simulink model "equations_PWSM"  (R2024b)
settings: Solver=VariableStepAuto  StartTime=0.0  StopTime=10.0  RelTol=1e-3
undefined symbols (not defined in the file): B, flux, J, Ld, Lq, pn, Pn, R
settings Model: Creator=罗芳成  LastModifiedBy=罗芳成

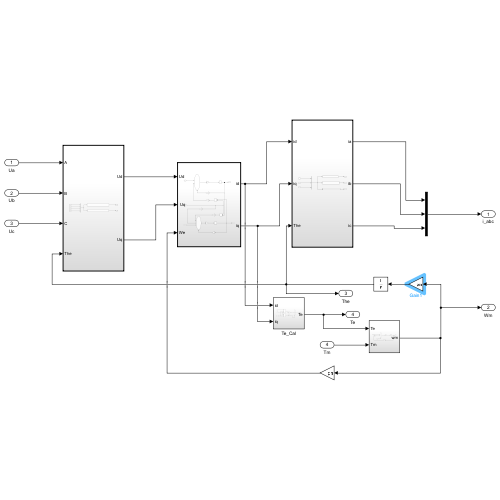
[thumbnail: Simulink's stored preview of the top-level diagram]
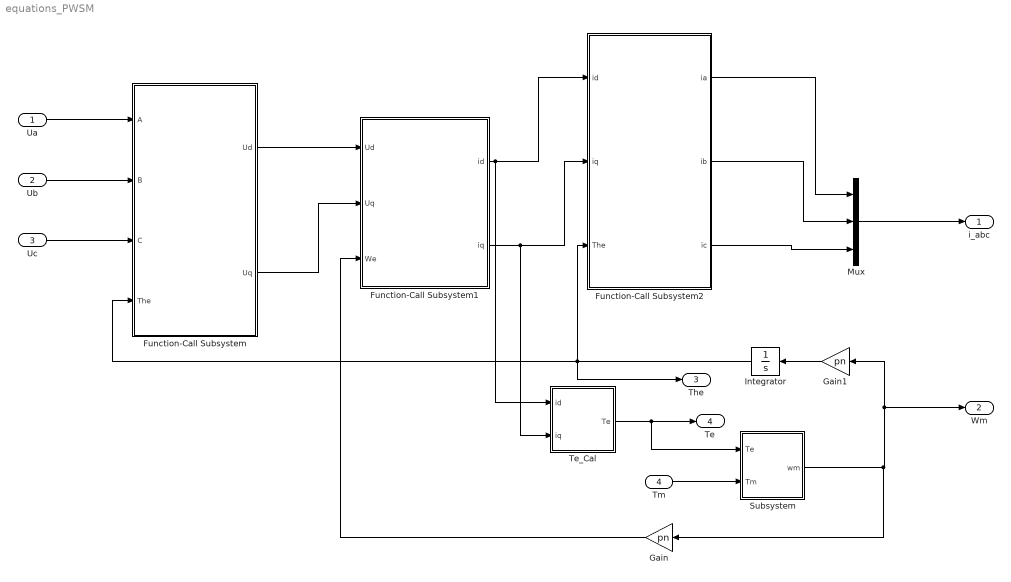
== system equations_PWSM ==
  Ua : Inport
  Ub : Inport  Port=2
  Uc : Inport  Port=3
  Tm : Inport  Port=4
  Function-Call Subsystem : Subsystem  TreatAsAtomicUnit=on
  Function-Call Subsystem1 : Subsystem  TreatAsAtomicUnit=on
  Function-Call Subsystem2 : Subsystem  TreatAsAtomicUnit=on
  Gain : Gain  Gain=pn
  Gain1 : Gain  Gain=pn
  Integrator : Integrator
  Mux : Mux  Inputs=3
  Subsystem : Subsystem
  Te_Cal : Subsystem
  i_abc : Outport
  Wm : Outport  Port=2
  The : Outport  Port=3
  Te : Outport  Port=4
  wires:
  Function-Call Subsystem2/1(ia) -> Mux/1
  Function-Call Subsystem2/2(ib) -> Mux/2
  Function-Call Subsystem2/3(ic) -> Mux/3
  Mux/1 -> i_abc/1
  Ua/1 -> Function-Call Subsystem/1(A)
  Ub/1 -> Function-Call Subsystem/2(B)
  Uc/1 -> Function-Call Subsystem/3(C)
  Function-Call Subsystem/1(Ud) -> Function-Call Subsystem1/1(Ud)
  Function-Call Subsystem/2(Uq) -> Function-Call Subsystem1/2(" Uq")
  Function-Call Subsystem1/1(id) -> Function-Call Subsystem2/1(id), Te_Cal/1(id)
  Function-Call Subsystem1/2(iq) -> Te_Cal/2(iq), Function-Call Subsystem2/2(iq)
  Te_Cal/1(Te) -> Subsystem/1(Te), Te/1
  Integrator/1 -> The/1, Function-Call Subsystem/4(The), Function-Call Subsystem2/3(The)
  Tm/1 -> Subsystem/2(Tm)
  Subsystem/1(wm) -> Gain/1, Gain1/1, Wm/1
  Gain/1 -> Function-Call Subsystem1/3(We)
  Gain1/1 -> Integrator/1

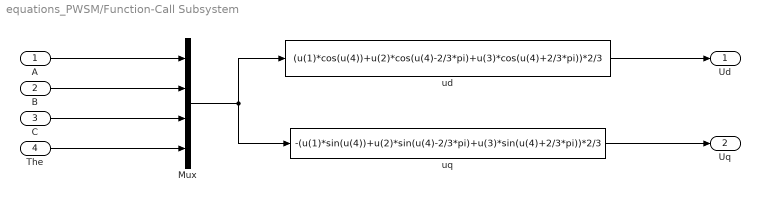
== system equations_PWSM/Function-Call Subsystem ==
  A : Inport
  B : Inport  Port=2
  C : Inport  Port=3
  The : Inport  Port=4
  Mux : Mux
  ud : Fcn  Expr=(u(1)*cos(u(4))+u(2)*cos(u(4)-2/3*pi)+u(3)*cos(u(4)+2/3*pi))*2/3
  uq : Fcn  Expr=-(u(1)*sin(u(4))+u(2)*sin(u(4)-2/3*pi)+u(3)*sin(u(4)+2/3*pi))*2/3
  Ud : Outport
  Uq : Outport  Port=2
  wires:
  uq/1 -> Uq/1
  The/1 -> Mux/4
  C/1 -> Mux/3
  Mux/1 -> uq/1, ud/1
  B/1 -> Mux/2
  A/1 -> Mux/1
  ud/1 -> Ud/1

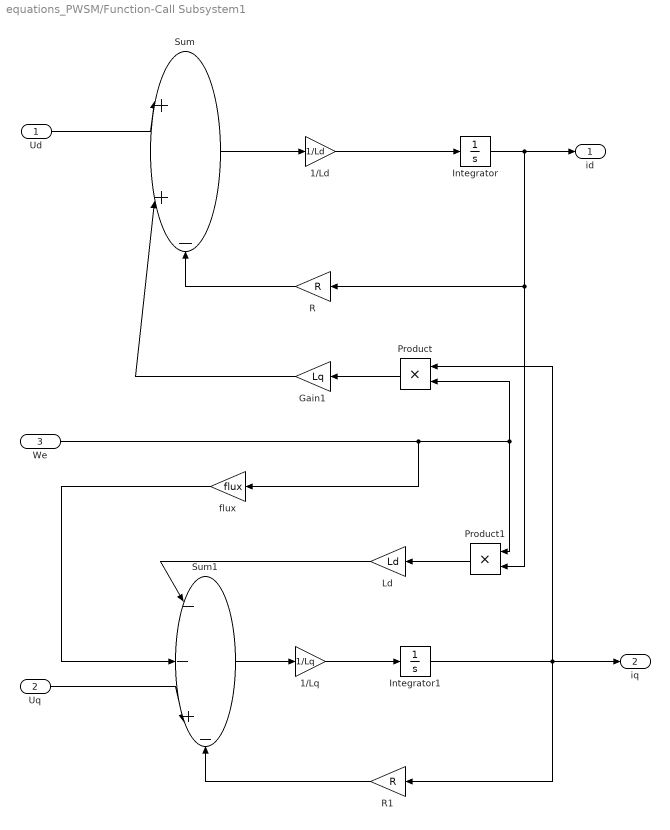
== system equations_PWSM/Function-Call Subsystem1 ==
  Ud : Inport
  " Uq" : Inport  Port=2
  We : Inport  Port=3
  1/Ld : Gain  Gain=1/Ld
  1/Lq : Gain  Gain=1/Lq
  Gain1 : Gain  Gain=Lq
  Integrator : Integrator
  Integrator1 : Integrator
  Ld : Gain  Gain=Ld
  Product : Product
  Product1 : Product
  R : Gain  Gain=R
  R1 : Gain  Gain=R
  Sum : Sum  Inputs=|++-
  Sum1 : Sum  Inputs=|--+-
  flux : Gain  Gain=flux
  id : Outport
  iq : Outport  Port=2
  wires:
  Ud/1 -> Sum/1
  Sum/1 -> 1/Ld/1
  1/Ld/1 -> Integrator/1
  Integrator/1 -> id/1, Product1/2, R/1
  R/1 -> Sum/3
  Product/1 -> Gain1/1
  Gain1/1 -> Sum/2
  " Uq"/1 -> Sum1/3
  flux/1 -> Sum1/2
  We/1 -> flux/1, Product1/1, Product/2
  Integrator1/1 -> R1/1, iq/1, Product/1
  Product1/1 -> Ld/1
  Ld/1 -> Sum1/1
  Sum1/1 -> 1/Lq/1
  1/Lq/1 -> Integrator1/1
  R1/1 -> Sum1/4

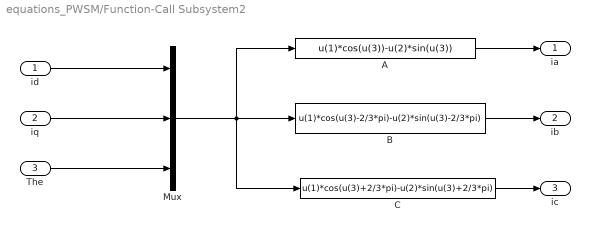
== system equations_PWSM/Function-Call Subsystem2 ==
  id : Inport
  iq : Inport  Port=2
  The : Inport  Port=3
  A : Fcn  Expr=u(1)*cos(u(3))-u(2)*sin(u(3))
  B : Fcn  Expr=u(1)*cos(u(3)-2/3*pi)-u(2)*sin(u(3)-2/3*pi)
  C : Fcn  Expr=u(1)*cos(u(3)+2/3*pi)-u(2)*sin(u(3)+2/3*pi)
  Mux : Mux  Inputs=3
  ia : Outport
  ib : Outport  Port=2
  ic : Outport  Port=3
  wires:
  id/1 -> Mux/1
  The/1 -> Mux/3
  Mux/1 -> C/1, A/1, B/1
  A/1 -> ia/1
  B/1 -> ib/1
  iq/1 -> Mux/2
  C/1 -> ic/1

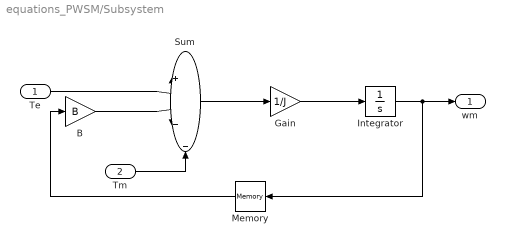
== system equations_PWSM/Subsystem ==
  Te : Inport
  Tm : Inport  Port=2
  B : Gain  Gain=B
  Gain : Gain  Gain=1/J
  Integrator : Integrator
  Memory : Memory
  Sum : Sum  Inputs=|+--
  wm : Outport
  wires:
  Te/1 -> Sum/1
  B/1 -> Sum/2
  Memory/1 -> B/1
  Tm/1 -> Sum/3
  Sum/1 -> Gain/1
  Gain/1 -> Integrator/1
  Integrator/1 -> wm/1, Memory/1

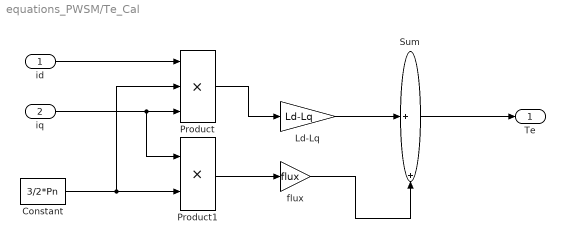
== system equations_PWSM/Te_Cal ==
  id : Inport
  iq : Inport  Port=2
  Constant : Constant  Value=3/2*Pn
  Ld-Lq : Gain  Gain=Ld-Lq
  Product : Product  Inputs=3
  Product1 : Product
  Sum : Sum  Inputs=|++
  flux : Gain  Gain=flux
  Te : Outport
  wires:
  id/1 -> Product/1
  iq/1 -> Product1/1, Product/3
  Constant/1 -> Product/2, Product1/2
  Product1/1 -> flux/1
  Product/1 -> Ld-Lq/1
  Ld-Lq/1 -> Sum/1
  flux/1 -> Sum/2
  Sum/1 -> Te/1
